simulink model "blockdiag"  (Simulink 3.00)
settings: Solver=ode45  SolverMode=SingleTasking  StartTime=0.0  StopTime=10.0  RelTol=1e-3  AbsTol=1e-6
undefined symbols (not defined in the file): C, L, R
settings Model: LastModifiedBy=eechris

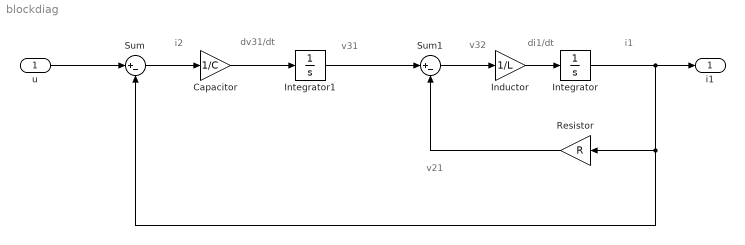
== system blockdiag ==
  note: dv31/dt
  note: v31
  note: v32
  note: di1/dt
  note: i1
  note: v21
  note: i2
  u : Inport  Port=1  PortWidth=-1  SampleTime=-1  DataType=auto
      settings: SignalType=auto
  Capacitor : Gain  Gain=1/C  SaturateOnIntegerOverflow=off
  Inductor : Gain  Gain=1/L  SaturateOnIntegerOverflow=on
  Integrator : Integrator  ExternalReset=none  InitialConditionSource=internal  InitialCondition=0  LimitOutput=off  UpperSaturationLimit=inf  LowerSaturationLimit=-inf  ShowSaturationPort=off  ShowStatePort=off  AbsoluteTolerance=auto
  Integrator1 : Integrator  ExternalReset=none  InitialConditionSource=internal  InitialCondition=0  LimitOutput=off  UpperSaturationLimit=inf  LowerSaturationLimit=-inf  ShowSaturationPort=off  ShowStatePort=off  AbsoluteTolerance=auto
  Resistor : Gain  Orientation=left  Gain=R  SaturateOnIntegerOverflow=on
  Sum : Sum  Inputs=|+-  SaturateOnIntegerOverflow=off
  Sum1 : Sum  Inputs=|+-  SaturateOnIntegerOverflow=off
  i1 : Outport  Port=1
  wires:
  Inductor/1 -> Integrator/1
  Sum1/1 -> Inductor/1
  Capacitor/1 -> Integrator1/1
  Sum/1 -> Capacitor/1
  Integrator/1 -> Resistor/1, Sum/2, i1/1
  u/1 -> Sum/1
  Integrator1/1 -> Sum1/1
  Resistor/1 -> Sum1/2
